simulink model "Project_4_Simulink_Update"  (R2023b)
settings: Solver=VariableStepAuto  StartTime=0.0  StopTime=130  FixedStep=0.1  MinStep=0.1  RelTol=1e-3
values from neighbouring files (symbols this model uses):
  A = 2.32    [P4init.m]    (also in init.m)
  C_lambda_norm = 0    [P4init.m]    (also in init.m)
  Cd = 0.36    [P4init.m]    (also in init.m)
  DriveData = HighwayDriveData    [(Ignore)Project_4_matcode_updated.m]    (also in P4_new_matcode.m; p4_runsim.m)
  eta = 0.001    [P4init.m]    (also in init.m)
  g = 9.81    [P4init.m]    (also in init.m)
  init_theta_ddot = 0    [P4init.m]    (also in init.m)
  init_theta_dot = 0    [P4init.m]    (also in init.m)
  mph2mps = 1600/3600    (= 0.444444444444)    [P4init.m]    (also in init.m)
  mu = 1    [P4init.m]    (also in init.m)
  mu_b = 1    [P4init.m]    (also in init.m)
  Nb_max = 10000    [P4init.m]    (also in init.m)
  Rho = 1.225    [P4init.m]    (also in init.m)
  rps2rpm = 60/(2*pi())    [P4init.m]    (also in init.m)
  Time = HighwayTime    [(Ignore)Project_4_matcode_updated.m]    (also in P4_new_matcode.m; p4_runsim.m)
  vw = 0    [P4init.m]    (also in init.m)
  Wp = [transpose(x), transpose(y)]    [(Ignore)Project_4_matcode_updated.m]    (also in P4_new_matcode.m; P4_runsim.m; p4_new_matcode.m)
undefined symbols (not defined in the file or in its folder): batData, carData, motorData
libraries: slpidlib x2, simulink x1
settings Model: Creator=mbfia  LastModifiedBy=colby
settings DataIOCC: SaveState=on

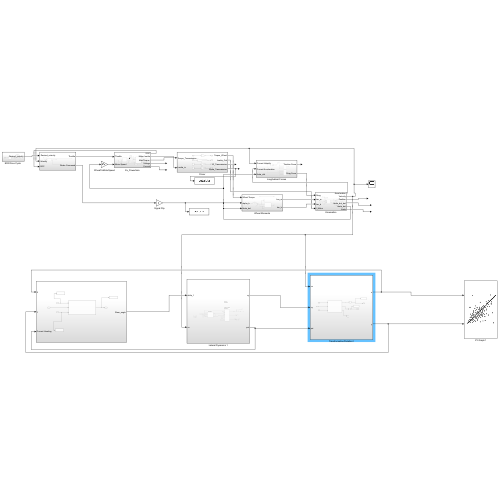
[thumbnail: Simulink's stored preview of the top-level diagram]
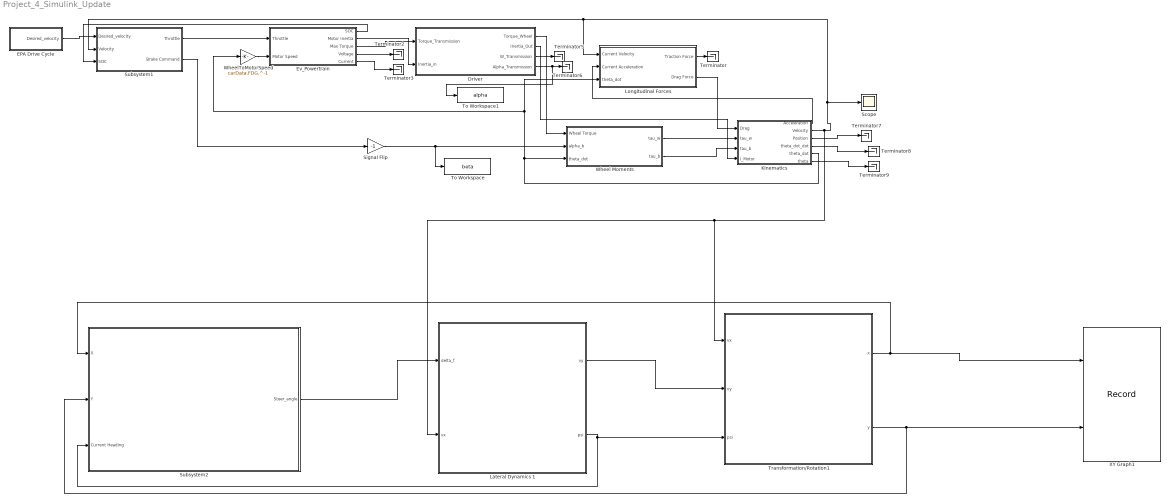
== system Project_4_Simulink_Update ==
  Driver : Subsystem
  "EPA Drive Cycle " : Subsystem
  Ev_Powertrain : Subsystem
  Kinematics : Subsystem
  Lateral Dynamics 1 : Subsystem
  Longitudinal Forces : Subsystem
  Scope : Scope
  Signal Flip : Gain  Gain=-1
  Subsystem1 : Subsystem
  Subsystem2 : Subsystem
  Terminator{,2..3,5..9} (8 alike) : Terminator
  To Workspace : ToWorkspace  VariableName=beta  SaveFormat=Timeseries  SampleTime=-1
  To Workspace1 : ToWorkspace  VariableName=alpha  SaveFormat=Timeseries  SampleTime=-1
  Transformation/Rotation1 : Subsystem
  Wheel Moments : Subsystem
  WheelToMotorSpeed : Gain  Gain=carData.FDG.^-1
  XY Graph1 : Record  FileSettingsInternal="{\"entries\":[{\"content\":{\"excelSettings\":{\"content\":{},\"type\":\"Streamout.ExcelSettings\"}},\"type\":\"Streamout.FileSettingStorage\",\"uuid\":\"\"}],\"packageUris\":[\"http:\\/\\/schema.mathworks.com\\/mf0\\/streamout_blocks\\/R2020a\"],\"version\":\"1.0\"}"  Layout=[1 1]  SignalsInternal="{\"entries\":[{\"content\":{\"signals\":[{\"content\":{\"blockPath\":[],\"dimensions\":[1],\"domain\":\"\",\"lineColor\":\"#a2142f\",\"plots\":[1],\"port\":1,\"signalID\":17127,\"signalName\":\"Transformation\\/Rotation1:1\"},\"type\":\"RecordBlkView.Signal\",\"uuid\":\"\"},{\"content\":{\"blockPath\":[],\"dimensions\":[1],\"domain\":\"\",\"lineColor\":\"#139fff\",\"plots\":[1],\"port\":2,\"signalID\":17130,\"signalName\":\"Transformation\\/Rotation1:2\"},\"type\":\"RecordBlkView.Signal\",\"uuid\":\"\"}]},\"type\":\"RecordBlkView.InputSignals\",\"uuid\":\"\"}],\"packageUris\":[\"http:\\/\\/schema.mathworks.com\\/mf0\\/streamout_blocks\\/R2020a\"],\"version\":\"1.0\"}"  VisualizationBindings="{\"xyplotplugin\":{\"info\":[{\"series\":[{\"bindingParametersList\":[{\"parameter\":\"X-Axis\",\"signalID\":17127,\"signalName\":\"Transformation\\/Rotation1:1\"},{\"parameter\":\"Y-Axis\",\"signalID\":17130,\"signalName\":\"Transformation\\/Rotation1:2\"}],\"seriesID\":3259}],\"subplotID\":1}]}}"  CompatibilityTag=XY
  wires:
  Kinematics/2(Velocity) -> Transformation/Rotation1/1(vx), Lateral Dynamics 1/2(vx), Scope/1, Subsystem1/2(Velocity), Longitudinal Forces/1(Current Velocity)
  Kinematics/1(Acceleration) -> Longitudinal Forces/2(Current Acceleration)
  Kinematics/5(theta_dot) -> WheelToMotorSpeed/1, Longitudinal Forces/3(theta_dot), Wheel Moments/3(theta_dot)
  Wheel Moments/1(tau_w) -> Kinematics/2(tau_w)
  Wheel Moments/2(tau_b) -> Kinematics/3(tau_b)
  Longitudinal Forces/1(Traction Force) -> Terminator/1
  Ev_Powertrain/4(Voltage) -> Terminator2/1
  Ev_Powertrain/5(Current) -> Terminator3/1
  Ev_Powertrain/3("Max Torque ") -> Driver/1(Torque_Transmission)
  Ev_Powertrain/2(Motor Inertia) -> Driver/2(Inertia_in)
  Driver/1(Torque_Wheel) -> Wheel Moments/1(Wheel Torque)
  Driver/3(W_Transmission) -> Terminator5/1
  Driver/4(Alpha_Transmission) -> To Workspace1/1, Terminator6/1
  Kinematics/3(Position) -> Terminator7/1
  Kinematics/4(theta_dot_dot) -> Terminator8/1
  Kinematics/6(theta) -> Terminator9/1
  Driver/2(Inertia_Out) -> Kinematics/4(I_Motor)
  Signal Flip/1 -> To Workspace/1, Wheel Moments/2(alpha_b)
  Longitudinal Forces/2(Drag Force) -> Kinematics/1(Drag)
  WheelToMotorSpeed/1 -> Ev_Powertrain/2(Motor Speed)
  "EPA Drive Cycle "/1(Desired_velocity) -> Subsystem1/1(" Desired_velocity")
  Subsystem1/1(Throttle) -> Ev_Powertrain/1(Throttle)
  Subsystem1/2(Brake Command) -> Signal Flip/1
  Ev_Powertrain/1(SOC) -> Subsystem1/3(SOC)
  Lateral Dynamics 1/2(psi) -> Subsystem2/3(Current Heading), Transformation/Rotation1/3(psi)
  Subsystem2/1(Steer_angle) -> Lateral Dynamics 1/1(delta_f)
  Transformation/Rotation1/2(y) -> Subsystem2/2(Y), XY Graph1/2
  Transformation/Rotation1/1(x) -> Subsystem2/1(X), XY Graph1/1
  Lateral Dynamics 1/1(vy) -> Transformation/Rotation1/2(vy)

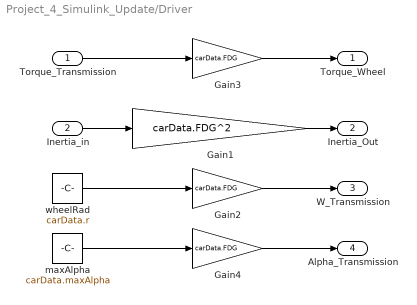
== system Project_4_Simulink_Update/Driver ==
  Torque_Transmission : Inport
  Inertia_in : Inport  Port=2
  Gain1 : Gain  Gain=carData.FDG^2
  Gain2 : Gain  Gain=carData.FDG
  Gain3 : Gain  Gain=carData.FDG
  Gain4 : Gain  Gain=carData.FDG
  maxAlpha : Constant  Value=carData.maxAlpha
  wheelRad : Constant  Value=carData.r
  Torque_Wheel : Outport
  Inertia_Out : Outport  Port=2
  W_Transmission : Outport  Port=3
  Alpha_Transmission : Outport  Port=4
  wires:
  Torque_Transmission/1 -> Gain3/1
  Gain3/1 -> Torque_Wheel/1
  Gain1/1 -> Inertia_Out/1
  Inertia_in/1 -> Gain1/1
  Gain2/1 -> W_Transmission/1
  wheelRad/1 -> Gain2/1
  Gain4/1 -> Alpha_Transmission/1
  maxAlpha/1 -> Gain4/1

== system Project_4_Simulink_Update/EPA Drive Cycle  ==
  1-D Lookup Table : Lookup_n-D  NumberOfTableDimensions=1  BreakpointsForDimension1=Time  Table=DriveData  InternalRulePriority=Speed  RndMeth=Simplest
  Clock : Clock
  Scope : Scope
  convert mph to m/s : Gain  Gain=mph2mps
  Desired_velocity : Outport
  wires:
  Clock/1 -> 1-D Lookup Table/1
  1-D Lookup Table/1 -> convert mph to m/s/1
  convert mph to m/s/1 -> Scope/1, Desired_velocity/1

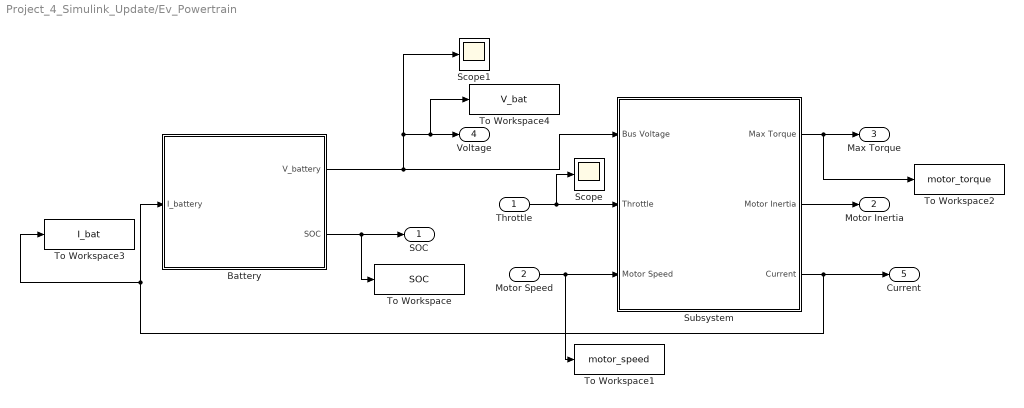
== system Project_4_Simulink_Update/Ev_Powertrain ==
  Throttle : Inport
  Motor Speed : Inport  Port=2
  Battery : Subsystem
  Scope : Scope
  Scope1 : Scope
  Subsystem : Subsystem
  To Workspace : ToWorkspace  VariableName=SOC  SaveFormat=Timeseries  SampleTime=-1
  To Workspace1 : ToWorkspace  VariableName=motor_speed  SaveFormat=Timeseries  SampleTime=-1
  To Workspace2 : ToWorkspace  VariableName=motor_torque  SaveFormat=Timeseries  SampleTime=-1
  To Workspace3 : ToWorkspace  VariableName=I_bat  SaveFormat=Timeseries  SampleTime=-1
  To Workspace4 : ToWorkspace  VariableName=V_bat  SaveFormat=Timeseries  SampleTime=-1
  SOC : Outport
  Motor Inertia : Outport  Port=2
  "Max Torque " : Outport  Port=3
  Voltage : Outport  Port=4
  Current : Outport  Port=5
  wires:
  Battery/2(SOC) -> To Workspace/1, SOC/1
  Battery/1(V_battery) -> Scope1/1, To Workspace4/1, Voltage/1, Subsystem/1(Bus Voltage)
  Throttle/1 -> Scope/1, Subsystem/2(Throttle)
  Motor Speed/1 -> To Workspace1/1, Subsystem/3(Motor Speed)
  Subsystem/3(Current) -> To Workspace3/1, Battery/1(I_battery), Current/1
  Subsystem/1("Max Torque ") -> To Workspace2/1, "Max Torque "/1
  Subsystem/2(Motor Inertia) -> Motor Inertia/1

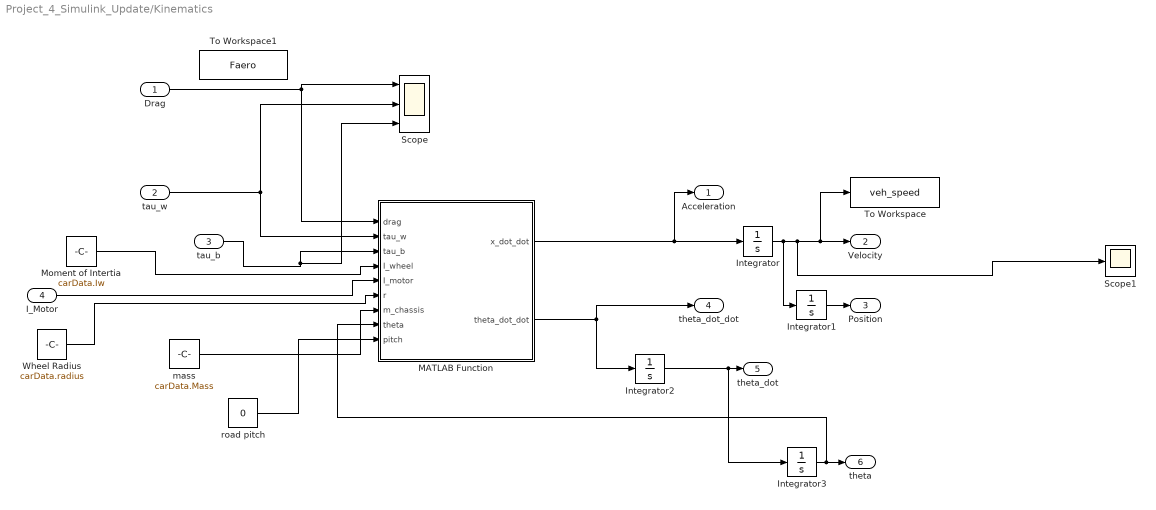
== system Project_4_Simulink_Update/Kinematics ==
  Drag : Inport
  tau_w : Inport  Port=2
  tau_b : Inport  Port=3
  I_Motor : Inport  Port=4
  Integrator : Integrator  InitialCondition=carData.init.vx0
  Integrator1 : Integrator  InitialCondition=carData.init.X0
  Integrator2 : Integrator  InitialCondition=init_theta_ddot
  Integrator3 : Integrator  InitialCondition=init_theta_dot
  MATLAB Function : MATLAB Function  TreatAsAtomicUnit=on
  Moment of Intertia : Constant  Value=carData.Iw
  Scope : Scope  NumInputPorts=3
  Scope1 : Scope
  To Workspace : ToWorkspace  VariableName=veh_speed  SaveFormat=Timeseries  SampleTime=-1
  To Workspace1 : ToWorkspace  VariableName=Faero  SaveFormat=Timeseries  SampleTime=-1
  Wheel Radius : Constant  Value=carData.radius
  mass : Constant  Value=carData.Mass
  road pitch : Constant  Value=0
  Acceleration : Outport
  Velocity : Outport  Port=2
  Position : Outport  Port=3
  theta_dot_dot : Outport  Port=4
  theta_dot : Outport  Port=5
  theta : Outport  Port=6
  wires:
  Integrator/1 -> Integrator1/1, Scope1/1, To Workspace/1, Velocity/1
  Integrator1/1 -> Position/1
  Drag/1 -> Scope/1, MATLAB Function/1(drag)
  mass/1 -> MATLAB Function/7(m_chassis)
  tau_w/1 -> Scope/2, MATLAB Function/2(tau_w)
  tau_b/1 -> Scope/3, MATLAB Function/3(tau_b)
  Moment of Intertia/1 -> MATLAB Function/4(I_wheel)
  Wheel Radius/1 -> MATLAB Function/6(r)
  MATLAB Function/1(x_dot_dot) -> Integrator/1, Acceleration/1
  MATLAB Function/2(theta_dot_dot) -> Integrator2/1, theta_dot_dot/1
  Integrator3/1 -> MATLAB Function/8(theta), theta/1
  Integrator2/1 -> Integrator3/1, theta_dot/1
  I_Motor/1 -> MATLAB Function/5(I_motor)
  road pitch/1 -> MATLAB Function/9(pitch)

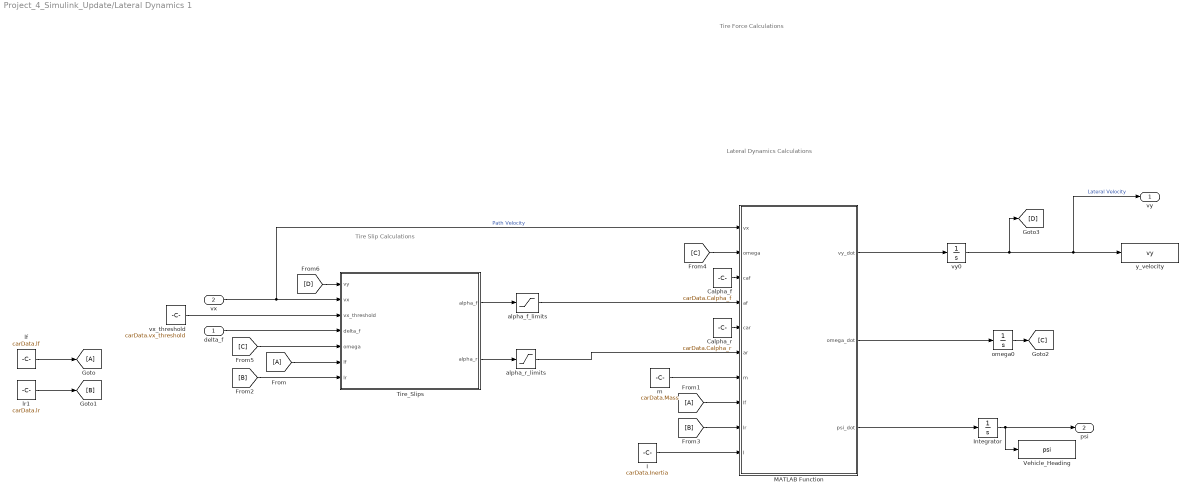
== system Project_4_Simulink_Update/Lateral Dynamics 1 ==
  note: Tire Slip Calculations
  note: Tire Force Calculations
  note: Lateral Dynamics Calculations
  delta_f : Inport
  vx : Inport  Port=2
  Calpha_f : Constant  Value=carData.Calpha_f
  Calpha_r : Constant  Value=carData.Calpha_r
  From : From
  From1 : From
  Goto : Goto
  I : Constant  Value=carData.Inertia
  Integrator : Integrator
  MATLAB Function : MATLAB Function  TreatAsAtomicUnit=on
  Tire_Slips : MATLAB Function  TreatAsAtomicUnit=on
  Vehicle_Heading : ToWorkspace  VariableName=psi  SaveFormat=Timeseries  SampleTime=-1
  alpha_f_limits : Saturate  UpperLimit=carData.maxAlpha  LowerLimit=-carData.maxAlpha
  alpha_r_limits : Saturate  UpperLimit=carData.maxAlpha  LowerLimit=-carData.maxAlpha
  lf : Constant  Value=carData.lf
  lr1 : Constant  Value=carData.lr
  m : Constant  Value=carData.Mass
  omega0 : Integrator  InitialCondition=carData.init.omega0
  vx_threshold : Constant  Value=carData.vx_threshold
  vy0 : Integrator  InitialCondition=carData.init.vy0
  y_velocity : ToWorkspace  VariableName=vy  SaveFormat=Timeseries  SampleTime=-1
  vy : Outport
  psi : Outport  Port=2
  wires:
  vx/1 -> Tire_Slips/2(vx), MATLAB Function/1(vx)  "Path Velocity"
  Tire_Slips/1(alpha_f) -> alpha_f_limits/1
  Tire_Slips/2(alpha_r) -> alpha_r_limits/1
  alpha_f_limits/1 -> MATLAB Function/4(af)
  alpha_r_limits/1 -> MATLAB Function/6(ar)
  vy0/1 -> [D], vy/1, y_velocity/1  "Lateral Velocity"
  delta_f/1 -> Tire_Slips/4(delta_f)
  Calpha_f/1 -> MATLAB Function/3(caf)
  vx_threshold/1 -> Tire_Slips/3(vx_threshold)
  Calpha_r/1 -> MATLAB Function/5(car)
  MATLAB Function/2(omega_dot) -> omega0/1
  MATLAB Function/1(vy_dot) -> vy0/1
  I/1 -> MATLAB Function/10(I)
  MATLAB Function/3(psi_dot) -> Integrator/1
  Integrator/1 -> Vehicle_Heading/1, psi/1
  m/1 -> MATLAB Function/7(m)
  lf/1 -> Goto/1
  From/1 -> Tire_Slips/6(lf)
  From1/1 -> MATLAB Function/8(lf)
  lr1/1 -> [B]
  [B] -> Tire_Slips/7(lr)
  [B] -> MATLAB Function/9(lr)
  omega0/1 -> [C]
  [C] -> MATLAB Function/2(omega)
  [C] -> Tire_Slips/5(omega)
  [D] -> Tire_Slips/1(vy)

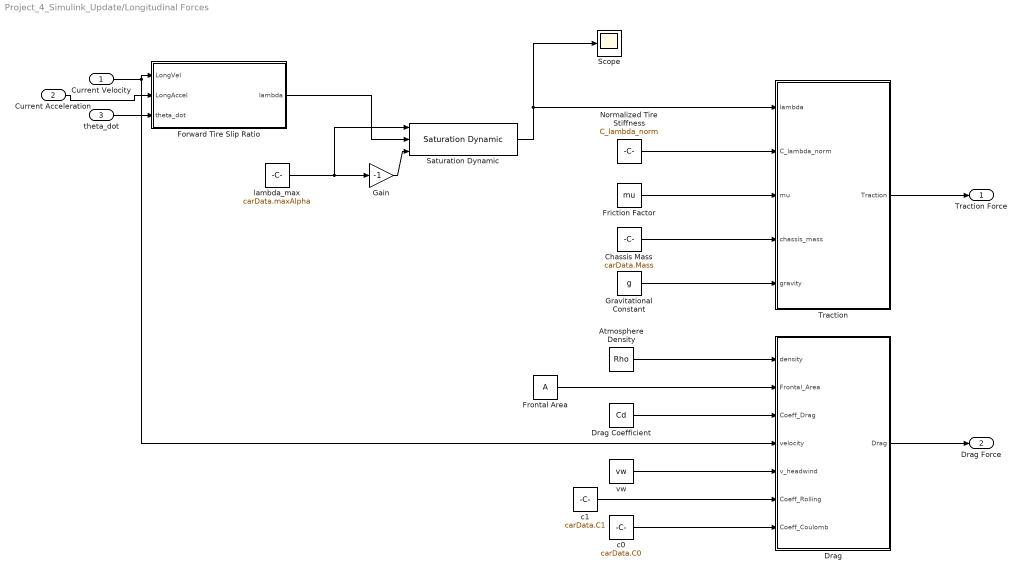
== system Project_4_Simulink_Update/Longitudinal Forces ==
  Current Velocity : Inport
  Current Acceleration : Inport  Port=2
  theta_dot : Inport  Port=3
  Atmosphere Density : Constant  Value=Rho
  Chassis Mass : Constant  Value=carData.Mass
  Drag : MATLAB Function  TreatAsAtomicUnit=on
  Drag Coefficient : Constant  Value=Cd
  Forward Tire Slip Ratio : Subsystem
  Friction Factor : Constant  Value=mu
  "Frontal Area " : Constant  Value=A
  Gain : Gain  Gain=-1
  Gravitational Constant : Constant  Value=g
  Normalized Tire Stiffness : Constant  Value=C_lambda_norm
  Saturation Dynamic : simulink/Discontinuities/Saturation Dynamic  OutMin=[]  OutMax=[]  OutDataTypeStr=Inherit: Same as second input  OutDataType=fixdt(1, 16)  OutScaling=2^-10  DoSatur=off
  Scope : Scope
  Traction : MATLAB Function  TreatAsAtomicUnit=on
  c0 : Constant  Value=carData.C0
  c1 : Constant  Value=carData.C1
  lambda_max : Constant  Value=carData.maxAlpha
  vw : Constant  Value=vw
  Traction Force : Outport
  Drag Force : Outport  Port=2
  wires:
  Current Velocity/1 -> Drag/4(velocity), Forward Tire Slip Ratio/1(LongVel)
  Current Acceleration/1 -> Forward Tire Slip Ratio/2(LongAccel)
  Forward Tire Slip Ratio/1(lambda) -> Saturation Dynamic/2
  Gain/1 -> Saturation Dynamic/3
  lambda_max/1 -> Gain/1, Saturation Dynamic/1
  Saturation Dynamic/1 -> Scope/1, Traction/1(lambda)
  Normalized Tire Stiffness/1 -> Traction/2(C_lambda_norm)
  Friction Factor/1 -> Traction/3(mu)
  Chassis Mass/1 -> Traction/4(chassis_mass)
  Gravitational Constant/1 -> Traction/5(gravity)
  "Frontal Area "/1 -> Drag/2(Frontal_Area)
  Atmosphere Density/1 -> Drag/1(density)
  Drag Coefficient/1 -> Drag/3(Coeff_Drag)
  vw/1 -> Drag/5(v_headwind)
  c0/1 -> Drag/7(Coeff_Coulomb)
  c1/1 -> Drag/6(Coeff_Rolling)
  theta_dot/1 -> Forward Tire Slip Ratio/3(theta_dot)
  Traction/1(Traction) -> Traction Force/1
  Drag/1(Drag) -> Drag Force/1

== system Project_4_Simulink_Update/Subsystem1 ==
  " Desired_velocity" : Inport
  Velocity : Inport  Port=2
  SOC : Inport  Port=3
  Acceleration Control : Subsystem
  To Workspace : ToWorkspace  VariableName=veh_speed_desd  SaveFormat=Timeseries  SampleTime=-1
  Throttle : Outport
  Brake Command : Outport  Port=2
  wires:
  Velocity/1 -> Acceleration Control/2(Velocity)
  Acceleration Control/1(Throttle) -> Throttle/1
  " Desired_velocity"/1 -> To Workspace/1, Acceleration Control/1(" Desired_velocity")
  Acceleration Control/2(Brake Command) -> Brake Command/1
  SOC/1 -> Acceleration Control/3(SOC)

== system Project_4_Simulink_Update/Subsystem2 ==
  X : Inport
  Y : Inport  Port=2
  Current Heading : Inport  Port=3
  Driver Input : Subsystem
  To Workspace : ToWorkspace  VariableName=X  SaveFormat=Timeseries  SampleTime=-1
  To Workspace1 : ToWorkspace  VariableName=Y  SaveFormat=Timeseries  SampleTime=-1
  To Workspace2 : ToWorkspace  VariableName=delta  SaveFormat=Timeseries  SampleTime=-1
  Steer_angle : Outport
  wires:
  Driver Input/1(steer_angle) -> To Workspace2/1, Steer_angle/1
  X/1 -> To Workspace/1, Driver Input/1(X)
  Y/1 -> To Workspace1/1, Driver Input/3(Y)
  Current Heading/1 -> Driver Input/2(vehicle_angle)

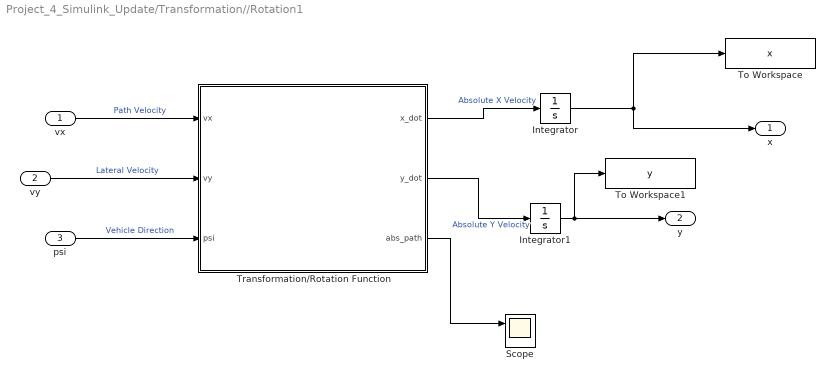
== system Project_4_Simulink_Update/Transformation//Rotation1 ==
  vx : Inport
  vy : Inport  Port=2
  psi : Inport  Port=3
  Integrator : Integrator
  Integrator1 : Integrator
  Scope : Scope  NumInputPorts=2
  To Workspace : ToWorkspace  VariableName=x  SaveFormat=Timeseries  SampleTime=-1
  To Workspace1 : ToWorkspace  VariableName=y  SaveFormat=Timeseries  SampleTime=-1
  Transformation/Rotation Function : MATLAB Function  TreatAsAtomicUnit=on
  x : Outport
  y : Outport  Port=2
  wires:
  vy/1 -> Transformation/Rotation Function/2(vy)  "Lateral Velocity"
  vx/1 -> Transformation/Rotation Function/1(vx)  "Path Velocity"
  psi/1 -> Transformation/Rotation Function/3(psi)  "Vehicle Direction"
  Transformation/Rotation Function/1(x_dot) -> Integrator/1  "Absolute X Velocity"
  Transformation/Rotation Function/2(y_dot) -> Integrator1/1  "Absolute Y Velocity"
  Integrator/1 -> x/1, To Workspace/1
  Integrator1/1 -> To Workspace1/1, y/1
  Transformation/Rotation Function/3(abs_path) -> Scope/1

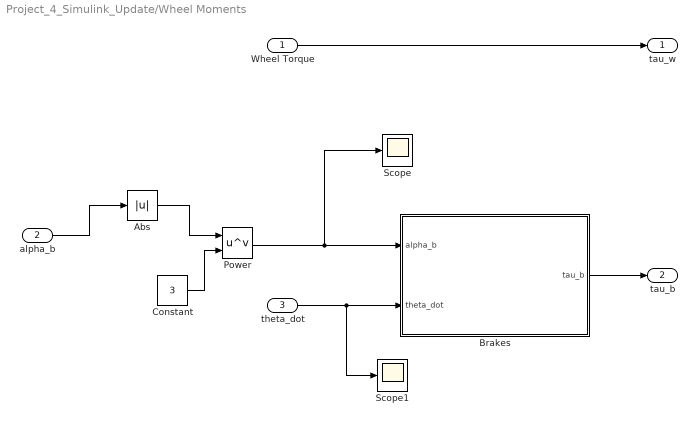
== system Project_4_Simulink_Update/Wheel Moments ==
  Wheel Torque : Inport
  alpha_b : Inport  Port=2
  theta_dot : Inport  Port=3
  Abs : Abs  SaturateOnIntegerOverflow=off
  Brakes : Subsystem
  Constant : Constant  Value=3
  Power : Math  Operator=pow
  Scope : Scope
  Scope1 : Scope
  tau_w : Outport
  tau_b : Outport  Port=2
  wires:
  theta_dot/1 -> Scope1/1, Brakes/2(theta_dot)
  Brakes/1(tau_b) -> tau_b/1
  Wheel Torque/1 -> tau_w/1
  Power/1 -> Scope/1, Brakes/1(alpha_b)
  Constant/1 -> Power/2
  alpha_b/1 -> Abs/1
  Abs/1 -> Power/1

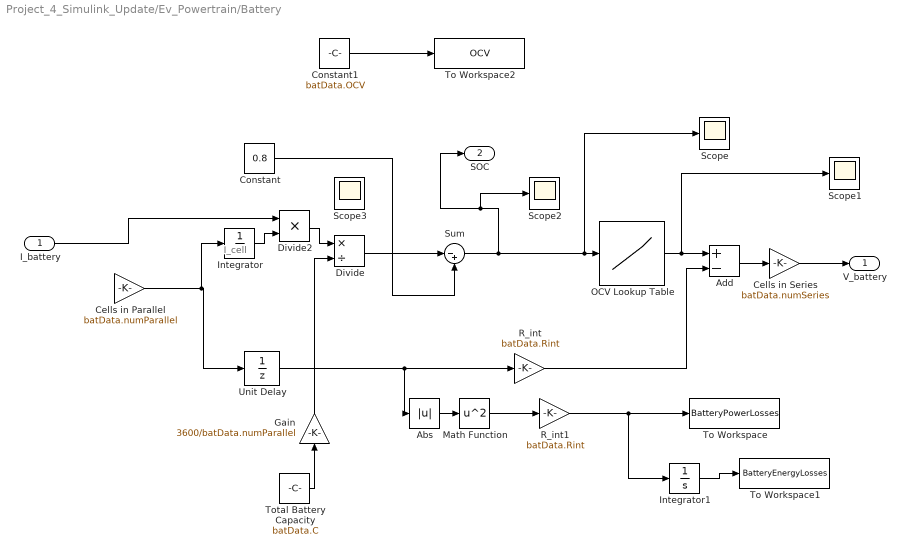
== system Project_4_Simulink_Update/Ev_Powertrain/Battery ==
  note: I_cell
  I_battery : Inport
  Abs : Abs  SaturateOnIntegerOverflow=off
  Add : Sum  Inputs=+-
  "Cells in Parallel " : Gain  Gain=batData.numParallel
  "Cells in Series " : Gain  Gain=batData.numSeries
  Constant : Constant  Value=0.8
  Constant1 : Constant  Value=batData.OCV
  Divide : Product  Inputs=*/
  Divide2 : Product  Inputs=**
  Gain : Gain  Gain=3600/batData.numParallel
  Integrator : Integrator
  Integrator1 : Integrator
  Math Function : Math  Operator=square
  OCV Lookup Table : Lookup_n-D  NumberOfTableDimensions=1  LookupTableObject=''  BreakpointsForDimension1=batData.SOC  BreakpointsForDimension2FirstPoint=10  BreakpointsForDimension1Spacing=12  BreakpointsForDimension2Spacing=12  Table=batData.OCV  InterpMethod=Flat  ExtrapMethod=Cubic spline  RemoveProtectionInput=on  InternalRulePriority=Speed  RndMeth=Simplest
  R_int : Gain  Gain=batData.Rint
  R_int1 : Gain  Gain=batData.Rint
  Scope{,1..3} (4 alike) : Scope
  Sum : Sum  Inputs=|-+
  To Workspace : ToWorkspace  VariableName=BatteryPowerLosses  SaveFormat=Timeseries  SampleTime=-1
  To Workspace1 : ToWorkspace  VariableName=BatteryEnergyLosses  SaveFormat=Timeseries  SampleTime=-1
  To Workspace2 : ToWorkspace  VariableName=OCV  SaveFormat=Timeseries  SampleTime=-1
  "Total Battery Capacity " : Constant  Value=batData.C
  Unit Delay : UnitDelay  SampleTime=-1  HasFrameUpgradeWarning=on
  V_battery : Outport
  SOC : Outport  Port=2
  wires:
  Divide/1 -> Sum/1
  Constant/1 -> Sum/2
  "Total Battery Capacity "/1 -> Gain/1
  Gain/1 -> Divide/2
  Unit Delay/1 -> Abs/1, R_int/1
  OCV Lookup Table/1 -> Scope1/1, Add/1
  R_int/1 -> Add/2
  Add/1 -> "Cells in Series "/1
  "Cells in Series "/1 -> V_battery/1
  Math Function/1 -> R_int1/1
  R_int1/1 -> Integrator1/1, To Workspace/1
  Integrator1/1 -> To Workspace1/1
  Sum/1 -> Scope/1, OCV Lookup Table/1, Scope2/1, SOC/1
  Constant1/1 -> To Workspace2/1
  Integrator/1 -> Divide2/2
  "Cells in Parallel "/1 -> Integrator/1, Unit Delay/1
  I_battery/1 -> Divide2/1
  Divide2/1 -> Divide/1
  Abs/1 -> Math Function/1

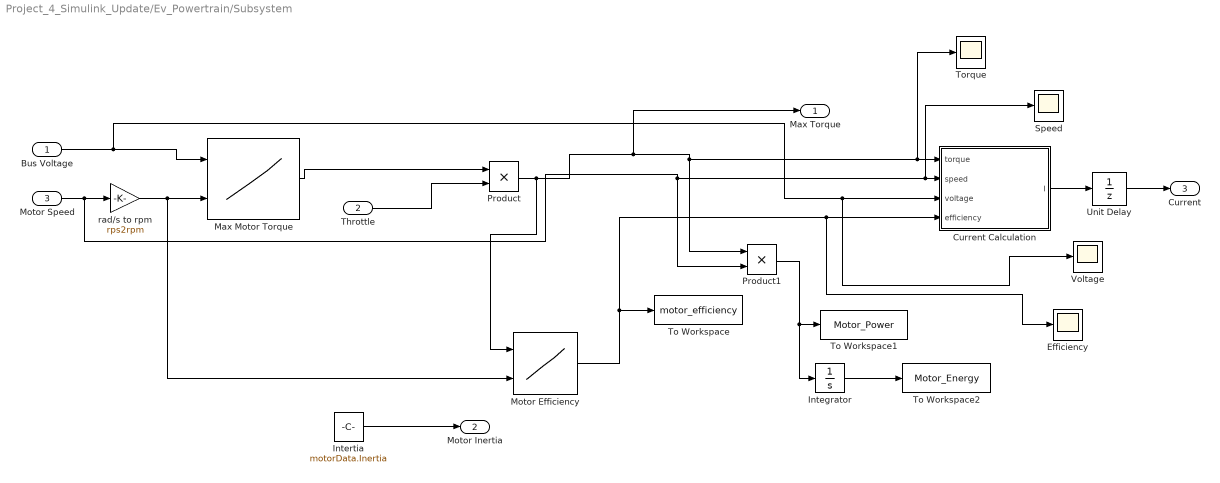
== system Project_4_Simulink_Update/Ev_Powertrain/Subsystem ==
  Bus Voltage : Inport
  Throttle : Inport  Port=2
  Motor Speed : Inport  Port=3
  "Current Calculation " : MATLAB Function  TreatAsAtomicUnit=on
  Efficiency : Scope
  Integrator : Integrator
  Intertia : Constant  Value=motorData.Inertia
  "Max Motor Torque " : Lookup_n-D  BreakpointsForDimension1=motorData.vbus  BreakpointsForDimension2=motorData.rpm  Table=motorData.maxtorque  InternalRulePriority=Speed  RndMeth=Simplest
      settings: InputPortMap=u0,u1
  Motor Efficiency : Lookup_n-D  BreakpointsForDimension1=motorData.eta_torque  BreakpointsForDimension2=motorData.eta_speed  Table=motorData.eta_val  InternalRulePriority=Speed  RndMeth=Simplest
      settings: InputPortMap=u0,u1
  Product : Product
  Product1 : Product
  Speed : Scope
  To Workspace : ToWorkspace  VariableName=motor_efficiency  SaveFormat=Timeseries  SampleTime=-1
  To Workspace1 : ToWorkspace  VariableName=Motor_Power  SaveFormat=Timeseries  SampleTime=-1
  To Workspace2 : ToWorkspace  VariableName=Motor_Energy  SaveFormat=Timeseries  SampleTime=-1
  Torque : Scope
  Unit Delay : UnitDelay  SampleTime=-1  HasFrameUpgradeWarning=on
  Voltage : Scope
  rad/s to rpm : Gain  Gain=rps2rpm
  "Max Torque " : Outport
  Motor Inertia : Outport  Port=2
  Current : Outport  Port=3
  wires:
  Motor Efficiency/1 -> To Workspace/1, "Current Calculation "/4(efficiency), Efficiency/1
  Throttle/1 -> Product/2
  Product/1 -> "Max Torque "/1, Product1/1, Torque/1, "Current Calculation "/1(torque), Motor Efficiency/1
  "Max Motor Torque "/1 -> Product/1
  Bus Voltage/1 -> "Current Calculation "/3(voltage), Voltage/1, "Max Motor Torque "/1
  Motor Speed/1 -> Product1/2, Speed/1, "Current Calculation "/2(speed), rad/s to rpm/1
  rad/s to rpm/1 -> Motor Efficiency/2, "Max Motor Torque "/2
  Intertia/1 -> Motor Inertia/1
  "Current Calculation "/1(I) -> Unit Delay/1
  Unit Delay/1 -> Current/1
  Product1/1 -> Integrator/1, To Workspace1/1
  Integrator/1 -> To Workspace2/1

== system Project_4_Simulink_Update/Longitudinal Forces/Forward Tire Slip Ratio ==
  LongVel : Inport
  LongAccel : Inport  Port=2
  theta_dot : Inport  Port=3
  MATLAB Function : MATLAB Function  TreatAsAtomicUnit=on
  Wheel Radius : Constant  Value=carData.radius
  lambda : Outport
  wires:
  MATLAB Function/1(lambda) -> lambda/1
  Wheel Radius/1 -> MATLAB Function/1(rw)
  LongVel/1 -> MATLAB Function/3(uw)
  LongAccel/1 -> MATLAB Function/4(accel)
  theta_dot/1 -> MATLAB Function/2(ww)

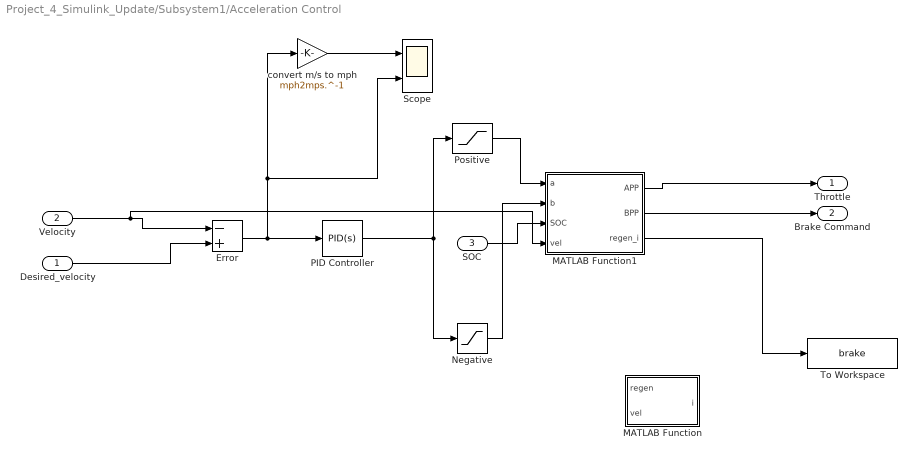
== system Project_4_Simulink_Update/Subsystem1/Acceleration Control ==
  " Desired_velocity" : Inport
  Velocity : Inport  Port=2
  SOC : Inport  Port=3
  Error : Sum  Inputs=-+
  MATLAB Function : MATLAB Function  TreatAsAtomicUnit=on
  MATLAB Function1 : MATLAB Function  TreatAsAtomicUnit=on
  Negative : Saturate  UpperLimit=0  LowerLimit=-1
  PID Controller : slpidlib/PID Controller  Controller=PID  Form=Parallel  TimeDomain=Continuous-time  UseExternalTs=off  SampleTime=-1  IntegratorMethod=Forward Euler  FilterMethod=Forward Euler  ControllerParametersSource=internal  P=0.57  I=0.03  UseKiTs=off  D=0  N=100  UseFilter=on  TunerSelectOption=Transfer Function Based (PID Tuner App)  InitialConditionSource=internal  InitialConditionForIntegrator=0  InitialConditionForFilter=0  DifferentiatorICPrevScaledInput=0  ExternalReset=none  TrackingMode=off  Kt=1  LimitOutput=off  SatLimitsSource=internal  UpperSaturationLimit=inf  LowerSaturationLimit=-inf  LinearizeAsGain=on  AntiWindupMode=none  Kb=1  LimitIntegrator=off  UpperIntegratorSaturationLimit=inf  LowerIntegratorSaturationLimit=-inf  POutMin=[]  POutMax=[]  IOutMin=[]  IOutMax=[]  DOutMin=[]  DOutMax=[]  NOutMin=[]  NOutMax=[]  SumOutMin=[]  SumOutMax=[]  SaturationOutMin=[]  SaturationOutMax=[]  PParamMin=[]  PParamMax=[]  IParamMin=[]  IParamMax=[]  DParamMin=[]  DParamMax=[]  NParamMin=[]  NParamMax=[]  KbParamMin=[]  KbParamMax=[]  KtParamMin=[]  KtParamMax=[]  KbOutMin=[]  KbOutMax=[]  KtOutMin=[]  KtOutMax=[]  IntegratorOutMin=[]  IntegratorOutMax=[]  FilterOutMin=[]  FilterOutMax=[]  SumI1OutMin=[]  SumI1OutMax=[]  SumI2OutMin=[]  SumI2OutMax=[]  SumI3OutMin=[]  SumI3OutMax=[]  SumI4OutMin=[]  SumI4OutMax=[]  SumDOutMin=[]  SumDOutMax=[]  DifferentiatorOutMin=[]  DifferentiatorOutMax=[]  FilterDiffOutCoefMin=[]  FilterDiffOutCoefMax=[]  ReciprocalOutMin=[]  ReciprocalOutMax=[]  SumDenOutMin=[]  SumDenOutMax=[]  SumNumOutMin=[]  SumNumOutMax=[]  DivideOutMin=[]  DivideOutMax=[]  UdiffTsProdOutMin=[]  UdiffTsProdOutMax=[]  NTsProdOutMin=[]  NTsProdOutMax=[]  UintegralTsProdOutMin=[]  UintegralTsProdOutMax=[]  UngainTsProdOutMin=[]  UngainTsProdOutMax=[]  ClampingZeroOutDataTypeStr=Inherit: Inherit via back propagation  ClampingZeroOutMin=[]  ClampingZeroOutMax=[]  FilterDenConstantOutDataTypeStr=Inherit: Inherit via back propagation  FilterDenConstantOutMin=[]  FilterDenConstantOutMax=[]  PCopyOutDataTypeStr=Inherit: Inherit via back propagation  PCopyOutMin=[]  PCopyOutMax=[]  NCopyOutDataTypeStr=Inherit: Inherit via back propagation  NCopyOutMin=[]  NCopyOutMax=[]  IntegratorContinuousStateAttributes=''  IntegratorStateMustResolveToSignalObject=off  IntegratorRTWStateStorageClass=Auto  FilterContinuousStateAttributes=''  FilterStateMustResolveToSignalObject=off  FilterRTWStateStorageClass=Auto  ParallelPVariant=InternalParameters  IdealPVariant=Disabled  IVariant=InternalParameters  DVariant=InternalParameters  IntegratorVariant=Continuous  SatVariant=Disabled  AWVariant=Passthrough  PCopyVariant=Disabled  TRVariant=Disabled  FdbkBlocksVariant=Forward  IdealPFdbkVariant=Disabled  SatFdbkVariant=Disabled  DerivativeFilterVariant=ContFilter  NVariant=InternalParameters  NCopyVariant=Disabled  FilterICVariant=InternalICsFilter  IntegratorICVariant=InternalICs  ExternalResetVariant=Disabled  TRSumVariant=Passthrough  SumFdbkVariant=Disabled  SumVariant=Sum_PID  TsampFilterVariant=InternalTs  TsampNgainVariant=Passthrough  TsampIntegralVariant=Disabled_SignalSpec  ExternalSaturationOutDataTypeStr=Inherit: Same as second input
  Positive : Saturate  UpperLimit=1  LowerLimit=0
  Scope : Scope  NumInputPorts=2
  To Workspace : ToWorkspace  VariableName=brake  SaveFormat=Timeseries  SampleTime=-1
  convert m/s to mph : Gain  Gain=mph2mps.^-1
  Throttle : Outport
  Brake Command : Outport  Port=2
  wires:
  Error/1 -> convert m/s to mph/1, Scope/2, PID Controller/1
  " Desired_velocity"/1 -> Error/2
  PID Controller/1 -> Positive/1, Negative/1
  convert m/s to mph/1 -> Scope/1
  Velocity/1 -> MATLAB Function1/4(vel), Error/1
  MATLAB Function1/1(APP) -> Throttle/1
  MATLAB Function1/2(BPP) -> Brake Command/1
  SOC/1 -> MATLAB Function1/3(SOC)
  Positive/1 -> MATLAB Function1/1(a)
  Negative/1 -> MATLAB Function1/2(b)
  MATLAB Function1/3(regen_i) -> To Workspace/1

== system Project_4_Simulink_Update/Subsystem2/Driver Input ==
  X : Inport
  vehicle_angle : Inport  Port=2
  Y : Inport  Port=3
  Calculate Error of Angle : MATLAB Function  TreatAsAtomicUnit=on
  Constant1 : Constant  Value=Wp
  Determine Target : MATLAB Function  TreatAsAtomicUnit=on
  Determine Target Direction : MATLAB Function  TreatAsAtomicUnit=on
  PID Controller : slpidlib/PID Controller  Controller=PID  Form=Parallel  TimeDomain=Continuous-time  UseExternalTs=off  SampleTime=-1  IntegratorMethod=Forward Euler  FilterMethod=Forward Euler  ControllerParametersSource=internal  P=1  I=0.1  UseKiTs=off  D=0  N=100  UseFilter=on  TunerSelectOption=Transfer Function Based (PID Tuner App)  InitialConditionSource=internal  InitialConditionForIntegrator=0  InitialConditionForFilter=0  DifferentiatorICPrevScaledInput=0  ExternalReset=none  TrackingMode=off  Kt=1  LimitOutput=off  SatLimitsSource=internal  UpperSaturationLimit=inf  LowerSaturationLimit=-inf  LinearizeAsGain=on  AntiWindupMode=none  Kb=1  LimitIntegrator=off  UpperIntegratorSaturationLimit=inf  LowerIntegratorSaturationLimit=-inf  POutMin=[]  POutMax=[]  IOutMin=[]  IOutMax=[]  DOutMin=[]  DOutMax=[]  NOutMin=[]  NOutMax=[]  SumOutMin=[]  SumOutMax=[]  SaturationOutMin=[]  SaturationOutMax=[]  PParamMin=[]  PParamMax=[]  IParamMin=[]  IParamMax=[]  DParamMin=[]  DParamMax=[]  NParamMin=[]  NParamMax=[]  KbParamMin=[]  KbParamMax=[]  KtParamMin=[]  KtParamMax=[]  KbOutMin=[]  KbOutMax=[]  KtOutMin=[]  KtOutMax=[]  IntegratorOutMin=[]  IntegratorOutMax=[]  FilterOutMin=[]  FilterOutMax=[]  SumI1OutMin=[]  SumI1OutMax=[]  SumI2OutMin=[]  SumI2OutMax=[]  SumI3OutMin=[]  SumI3OutMax=[]  SumI4OutMin=[]  SumI4OutMax=[]  SumDOutMin=[]  SumDOutMax=[]  DifferentiatorOutMin=[]  DifferentiatorOutMax=[]  FilterDiffOutCoefMin=[]  FilterDiffOutCoefMax=[]  ReciprocalOutMin=[]  ReciprocalOutMax=[]  SumDenOutMin=[]  SumDenOutMax=[]  SumNumOutMin=[]  SumNumOutMax=[]  DivideOutMin=[]  DivideOutMax=[]  UdiffTsProdOutMin=[]  UdiffTsProdOutMax=[]  NTsProdOutMin=[]  NTsProdOutMax=[]  UintegralTsProdOutMin=[]  UintegralTsProdOutMax=[]  UngainTsProdOutMin=[]  UngainTsProdOutMax=[]  ClampingZeroOutDataTypeStr=Inherit: Inherit via back propagation  ClampingZeroOutMin=[]  ClampingZeroOutMax=[]  FilterDenConstantOutDataTypeStr=Inherit: Inherit via back propagation  FilterDenConstantOutMin=[]  FilterDenConstantOutMax=[]  PCopyOutDataTypeStr=Inherit: Inherit via back propagation  PCopyOutMin=[]  PCopyOutMax=[]  NCopyOutDataTypeStr=Inherit: Inherit via back propagation  NCopyOutMin=[]  NCopyOutMax=[]  IntegratorContinuousStateAttributes=''  IntegratorStateMustResolveToSignalObject=off  IntegratorRTWStateStorageClass=Auto  FilterContinuousStateAttributes=''  FilterStateMustResolveToSignalObject=off  FilterRTWStateStorageClass=Auto  ParallelPVariant=InternalParameters  IdealPVariant=Disabled  IVariant=InternalParameters  DVariant=InternalParameters  IntegratorVariant=Continuous  SatVariant=Disabled  AWVariant=Passthrough  PCopyVariant=Disabled  TRVariant=Disabled  FdbkBlocksVariant=Forward  IdealPFdbkVariant=Disabled  SatFdbkVariant=Disabled  DerivativeFilterVariant=ContFilter  NVariant=InternalParameters  NCopyVariant=Disabled  FilterICVariant=InternalICsFilter  IntegratorICVariant=InternalICs  ExternalResetVariant=Disabled  TRSumVariant=Passthrough  SumFdbkVariant=Disabled  SumVariant=Sum_PID  TsampFilterVariant=InternalTs  TsampNgainVariant=Passthrough  TsampIntegralVariant=Disabled_SignalSpec  ExternalSaturationOutDataTypeStr=Inherit: Same as second input
  Subtract : Sum  Inputs=-+
  Subtract1 : Sum  Inputs=+-
  steer_angle : Outport
  wires:
  X/1 -> Subtract/1, Determine Target/1(X)
  Y/1 -> Subtract1/2, Determine Target/3(Y)
  Constant1/1 -> Determine Target/2(waypoints)
  Subtract/1 -> Determine Target Direction/1(dx)
  Subtract1/1 -> Determine Target Direction/2(dy)
  Determine Target/2(target_y) -> Subtract1/1
  Determine Target Direction/1(desired_angle) -> Calculate Error of Angle/1(target_angle)
  vehicle_angle/1 -> Calculate Error of Angle/2(current_angle)
  PID Controller/1 -> steer_angle/1
  Calculate Error of Angle/1(steer_angle) -> PID Controller/1
  Determine Target/1(target_x) -> Subtract/2

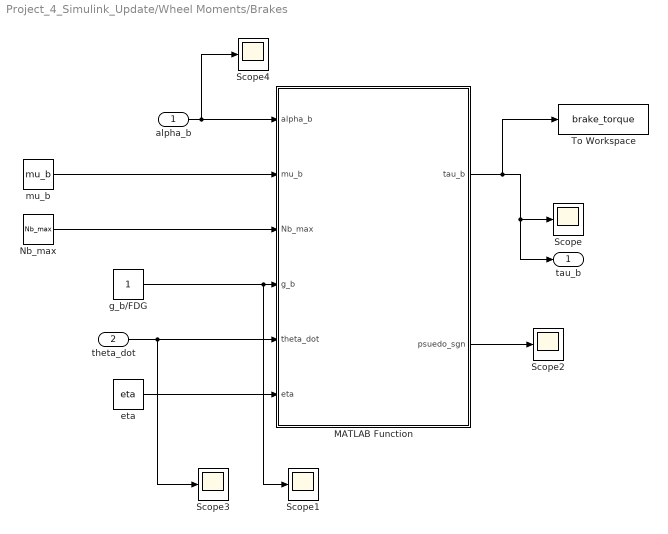
== system Project_4_Simulink_Update/Wheel Moments/Brakes ==
  alpha_b : Inport
  theta_dot : Inport  Port=2
  MATLAB Function : MATLAB Function  TreatAsAtomicUnit=on
  Nb_max : Constant  Value=Nb_max
  Scope{,1..4} (5 alike) : Scope
  To Workspace : ToWorkspace  VariableName=brake_torque  SaveFormat=Timeseries  SampleTime=-1
  eta : Constant  Value=eta
  g_b/FDG : Constant
  mu_b : Constant  Value=mu_b
  tau_b : Outport
  wires:
  alpha_b/1 -> Scope4/1, MATLAB Function/1(alpha_b)
  mu_b/1 -> MATLAB Function/2(mu_b)
  Nb_max/1 -> MATLAB Function/3(Nb_max)
  g_b/FDG/1 -> Scope1/1, MATLAB Function/4(g_b)
  theta_dot/1 -> Scope3/1, MATLAB Function/5(theta_dot)
  eta/1 -> MATLAB Function/6(eta)
  MATLAB Function/1(tau_b) -> To Workspace/1, tau_b/1, Scope/1
  MATLAB Function/2(psuedo_sgn) -> Scope2/1

== matlab function Project_4_Simulink_Update/Subsystem1/Acceleration Control/MATLAB Function1 ==
  data: a input; APP output; b input; SOC input; vel input; BPP output; regen_i output
function [APP, BPP, regen_i] = fcn(a, b, SOC, vel)

    % Convert velocity to m/s if it's provided in miles/hour
    vel_mps = vel * (1600/3600);
    
    % Define velocity thresholds
    vel_threshold_low = 5 * (1600/3600); % 5 mph in m/s
    vel_threshold_high = 25 * (1600/3600); % 25 mph in m/s
    
    % Define regenerative braking limits based on velocity
    if vel_mps < vel_threshold_low
        regen_i = 0;
    elseif vel_mps >= vel_threshold_low && vel_mps < vel_threshold_high
        % Linear interpolation between the thresholds
        regen_i = (0.95 / (vel_threshold_high - vel_threshold_low)) * (vel_mps - vel_threshold_low);
    else
        % Velocity is above the high threshold
        regen_i = 0.95;
    end

    % Check if the actual regen matches the expected regen_i
    if b > 0 % Only consider regen if there's a braking command
        regen = b; % Assume 'b' is the desired regen amount for simplicity
        if regen == regen_i
            i = 0;
        else
            i = 1;
        end
    else
        regen = 0;
        i = 0; % No regen if there's no braking command
    end
    
    % Calculate the Brake Pedal Position (BPP)
    BPP = regen; % Direct mapping for this example
    
    % Process acceleration command 'a'
    APP = a; % Assume 'a' is the desired APP amount for simplicity
    
    % Ensure APP and BPP do not conflict; zero APP if there's any regenerative braking
    if BPP > 0
        APP = 0;
    end

    % Ensure outputs are within allowable range
    APP = max(0, min(APP, 100));
    BPP = max(0, min(BPP, 100));

end

== matlab function Project_4_Simulink_Update/Lateral Dynamics 1/MATLAB Function ==
  data: vx input; vy_dot output; omega input; caf input; af input; car input; ar input; m input; lf input; lr input; omega_dot output; psi_dot output; I input
function [vy_dot, omega_dot, psi_dot] = calc_vy(vx, omega, caf, af, car, ar, m, lf, lr, I)

vy_dot = (caf * af + car * ar) / m - vx * omega;

omega_dot = (caf * af * lf - car*ar*lr) / I;

psi_dot = omega;

== matlab function Project_4_Simulink_Update/Lateral Dynamics 1/Tire_Slips ==
  data: vy input; alpha_f output; vx input; vx_threshold input; delta_f input; omega input; alpha_r output; lf input; lr input
function [alpha_f, alpha_r] = fcn(vy, vx, vx_threshold,delta_f, omega, lf, lr)

% INPUTS
% vy - Lateral velocity due to slip
% vx - Path velocity (forward velocity)
% delta_f - Angle of wheels due to steering (left/right) Radians
% omega - rate of yaw


% OUTPUTS
% alpha_f - Angle of slip for front tires (radians)
% alpha_r - Angle of slip for rear tires (radians)

if abs(vx) > vx_threshold
    alpha_f = angdiff((vy + lf * omega) / vx, delta_f); 
    alpha_r = - (vy - lr * omega) / vx; 
else
    alpha_f = 0;
    alpha_r = 0;
end

== matlab function Project_4_Simulink_Update/Subsystem2/Driver Input/Calculate Error of Angle ==
  data: target_angle input; steer_angle output; current_angle input
function steer_angle = diff(target_angle, current_angle)

steer_angle = angdiff(current_angle, target_angle);

== matlab function Project_4_Simulink_Update/Subsystem2/Driver Input/Determine Target ==
  data: X input; waypoints input; Y input; target_x output; target_y output
function [target_x, target_y] = Driver(X, waypoints, Y)

waypoints = waypoints(1:end-1,:);

% Determine which waypoint is the closest
dist_from_waypoints_sqr = (waypoints(:,1)-X).^2+(waypoints(:,2)-Y).^2;
dist_from_waypoints = sqrt(dist_from_waypoints_sqr);

[~, idx] = min(dist_from_waypoints);

% Look ahead a few waypoints
target_idx = idx + 2;
if target_idx >= height(waypoints)
   target_idx = 1;
end
target_x = waypoints(target_idx,1);
target_y = waypoints(target_idx,2);

== matlab function Project_4_Simulink_Update/Subsystem2/Driver Input/Determine Target Direction ==
  data: dx input; desired_angle output; dy input
function desired_angle = fcn(dx,dy)

desired_angle = atan2(dy,dx);

% Make desired_angle a positive value always
if desired_angle < 0
    desired_angle = desired_angle + 2 * pi;
end

== matlab function Project_4_Simulink_Update/Transformation//Rotation1/Transformation//Rotation Function ==
  data: vx input; x_dot output; vy input; psi input; y_dot output; abs_path output
function [x_dot,y_dot, abs_path] = fcn(vx, vy, psi)
% INPUTS
% vx - Path velocity (forward velocity)
% vy - Lateral velocity (side to side due to slip)
% psi - Vehicle heading (direction vehicle is pointing, radians)

% This function assumes that psi is given in radians. If using an input in
% degrees, be sure to use deg2rad()

R = [cos(psi), -sin(psi);
     sin(psi), cos(psi)];

% Perform the rotation using rotation matrix
rotated_coords = R * [vx;
                      vy];

abs_path = vx.^2 + vy.^2;

% OUTPUTS
x_dot = rotated_coords(1,:); % Velocity in x in absolute coordinates
y_dot = rotated_coords(2,:); % Velocity in y in absolute coordinates

== matlab function Project_4_Simulink_Update/Longitudinal Forces/Drag ==
  data: density input; Drag output; Frontal_Area input; Coeff_Drag input; velocity input; v_headwind input; Coeff_Rolling input; Coeff_Coulomb input
function Drag = fcn(density, Frontal_Area, Coeff_Drag, velocity, ...
    v_headwind, Coeff_Rolling, Coeff_Coulomb)

c0 = Coeff_Coulomb;

if velocity < 0
    c0 = -c0;
end

c1 = Coeff_Rolling;

c2 = 1/2 * density * Frontal_Area * Coeff_Drag;

Drag = c0 * + c1 * velocity + c2 * (velocity + v_headwind) .^ 2;

== matlab function Project_4_Simulink_Update/Longitudinal Forces/Traction ==
  data: Traction output; lambda input; C_lambda_norm input; mu input; chassis_mass input; gravity input
function Traction = fcn(lambda, C_lambda_norm, mu, chassis_mass, gravity)

N = chassis_mass * gravity;

C_lambda = C_lambda_norm * mu * N * lambda;

Traction = C_lambda * lambda;

== matlab function Project_4_Simulink_Update/Wheel Moments/Brakes/MATLAB Function ==
  data: alpha_b input; tau_b output; mu_b input; Nb_max input; g_b input; theta_dot input; eta input; psuedo_sgn output
function [tau_b, psuedo_sgn]= fcn(alpha_b, mu_b, Nb_max, g_b, theta_dot, eta)

psuedo_sgn = theta_dot / (abs(theta_dot)+ eta);

Nb = Nb_max * alpha_b;

tau_b = mu_b * Nb * g_b * psuedo_sgn;

== matlab function Project_4_Simulink_Update/Kinematics/MATLAB Function ==
  data: drag input; x_dot_dot output; tau_w input; tau_b input; I_wheel input; I_motor input; r input; m_chassis input; theta_dot_dot output; theta input; pitch input
function [x_dot_dot, theta_dot_dot]= fcn(drag, tau_w, tau_b, I_wheel, I_motor, r, m_chassis, theta, pitch)

Net_inertia = (I_wheel + I_motor) / r .^ 2 + m_chassis;


x_dot_dot = 1/Net_inertia * ( ...
    (tau_w - tau_b)/r - drag - (m_chassis * 9.81 * sin(pitch))...
    );





theta_dot_dot = x_dot_dot / r;

== matlab function Project_4_Simulink_Update/Longitudinal Forces/Forward Tire Slip Ratio/MATLAB Function ==
  data: rw input; lambda output; ww input; uw input; accel input
function lambda = fcn(rw, ww, uw, accel)

if accel >= 0
    lambda = (rw * ww - uw) / (rw * ww);
else
    lambda = (rw * ww - uw) / uw;
end

== matlab function Project_4_Simulink_Update/Ev_Powertrain/Subsystem/Current Calculation  ==
  data: torque input; speed input; voltage input; efficiency input; I output
function I = fcn(torque, speed, voltage, efficiency)
    Pm = torque * speed; % Mechanical power

    % Determine the sign of Pm, strictly +1 or -1
    if Pm >= 0
        sgn_m = 1;
    else
        sgn_m = -1;
    end

    % Calculate electrical power using the sign of mechanical power
    Pe = Pm * (efficiency ^ sgn_m);

    % Compute current
    I = Pe / voltage;
end

== matlab function Project_4_Simulink_Update/Subsystem1/Acceleration Control/MATLAB Function ==
  data: regen input; i output; vel input
function i = fcn(regen, vel)
    if vel < (5 * (1600/3600))
        regen_i = 0;
        if regen == regen_i
            i = 0;
        else
            i = 1;
        end
    
    elseif vel == (25 * (1600/3600))
        regen_i = 0.95;
        if regen == regen_i
            i = 0;
        else
            i = 1;
        end
    
    elseif vel > (25 * (1600/3600))
        regen_i = 0.95;
        if regen == regen_i
            i = 0;
        else
            i = 1;
        end
    else
        regen_i = (0.95/20) * vel;
        if regen == regen_i
            i = 0;
        else
            i = 1;
        end 
    end
